simulink model "invertedPendolum"  (R2019a)
settings: Solver=VariableStepAuto  StartTime=0.0  StopTime=60  FixedStep=0.0001  RelTol=1e-4
InitFcn:
  | simulationVar
values from neighbouring files (symbols this model uses):
  tauMotMax = Ka * Id    (= 55296484.32)    [simulationVar.m]
libraries: simulink x6
settings Model: Creator=alfyhack  LastModifiedBy=alfyhack
settings SolverCC: AlgebraicLoopSolver=LineSearch
settings DebuggingCC: UnderSpecifiedDimensionMsg=warning

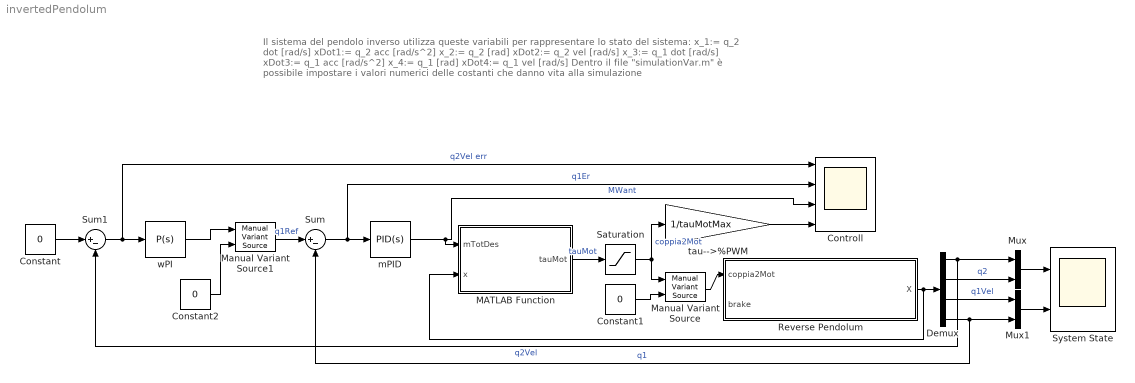
== system invertedPendolum ==
  note: Il sistema del pendolo inverso utilizza queste variabili per rappresentare lo stato del sistema:
      |
      | x_1:= q_2 dot  [rad/s]		xDot1:= q_2 acc   [rad/s^2]
      | x_2:= q_2        [rad]		xDot2:= q_2 vel    [rad/s]
      | x_3:= q_1 dot  [rad/s]		xDot3:= q_1 acc   [rad/s^2]
      | x_4:= q_1        [rad]		xDot4:= q_1 vel    [rad/s]
      |
      | Dentro il file "simulationVar.m" è possibile impostare i valori numerici delle costanti che danno vita alla simulazione
  Constant : Constant  Value=0
  Constant1 : Constant  Value=0
  Constant2 : Constant  Value=0
  Controll : Scope  NumInputPorts=4
  Demux : Demux
  MATLAB Function : MATLAB Function  TreatAsAtomicUnit=on
  Manual Variant Source : simulink/Signal Routing/Manual Variant Source  NumChoices=2  LabelModeActiveChoice=V_2
      settings: SourceProductName=Simulink
  Manual Variant Source1 : simulink/Signal Routing/Manual Variant Source  NumChoices=2  LabelModeActiveChoice=V_1
      settings: SourceProductName=Simulink
  Mux : Mux  Inputs=2
  Mux1 : Mux  Inputs=2
  Reverse Pendolum : Subsystem
  Saturation : Saturate  UpperLimit=tauMotMax  LowerLimit=-tauMotMax
  Sum : Sum  Inputs=|+-
  Sum1 : Sum  Inputs=|+-
  System State : Scope  NumInputPorts=2
  mPID : simulink/Continuous/PID Controller  Controller=PID  Form=Parallel  TimeDomain=Continuous-time  SampleTime=-1  IntegratorMethod=Forward Euler  FilterMethod=Forward Euler  ControllerParametersSource=internal  P=2418132733.30145  I=2565122053.15996  D=559751835.250899  UseFilter=on  N=123.582703784114  TunerSelectOption=Transfer Function Based (PID Tuner App)  InitialConditionSource=internal  InitialConditionForIntegrator=0  InitialConditionForFilter=0  DifferentiatorICPrevScaledInput=0  ExternalReset=none  TrackingMode=off  Kt=1  LimitOutput=off  UpperSaturationLimit=1000  LowerSaturationLimit=1000  LinearizeAsGain=off  AntiWindupMode=none  Kb=1  POutMin=[]  POutMax=[]  IOutMin=[]  IOutMax=[]  DOutMin=[]  DOutMax=[]  NOutMin=[]  NOutMax=[]  SumOutMin=[]  SumOutMax=[]  SaturationOutMin=[]  SaturationOutMax=[]  PParamMin=[]  PParamMax=[]  IParamMin=[]  IParamMax=[]  DParamMin=[]  DParamMax=[]  NParamMin=[]  NParamMax=[]  KbParamMin=[]  KbParamMax=[]  KtParamMin=[]  KtParamMax=[]  KbOutMin=[]  KbOutMax=[]  KtOutMin=[]  KtOutMax=[]  IntegratorOutMin=[]  IntegratorOutMax=[]  FilterOutMin=[]  FilterOutMax=[]  SumI1OutMin=[]  SumI1OutMax=[]  SumI2OutMin=[]  SumI2OutMax=[]  SumI3OutMin=[]  SumI3OutMax=[]  SumI4OutMin=[]  SumI4OutMax=[]  SumDOutMin=[]  SumDOutMax=[]  DifferentiatorOutMin=[]  DifferentiatorOutMax=[]  FilterDiffOutCoefMin=[]  FilterDiffOutCoefMax=[]  ReciprocalOutMin=[]  ReciprocalOutMax=[]  SumDenOutMin=[]  SumDenOutMax=[]  SumNumOutMin=[]  SumNumOutMax=[]  DivideOutMin=[]  DivideOutMax=[]  IntegratorContinuousStateAttributes=''  IntegratorStateMustResolveToSignalObject=off  IntegratorRTWStateStorageClass=Auto  FilterContinuousStateAttributes=''  FilterStateMustResolveToSignalObject=off  FilterRTWStateStorageClass=Auto  ParallelPVariant=InternalParameters  IdealPVariant=Disabled  IVariant=InternalParameters  DVariant=InternalParameters  IntegratorVariant=Continuous  SatVariant=Disabled  AWVariant=Passthrough  PCopyVariant=Disabled  TRVariant=Disabled  FdbkBlocksVariant=Forward  IdealPFdbkVariant=Disabled  SatFdbkVariant=Disabled  DerivativeFilterVariant=ContFilter  NVariant=InternalParameters  NCopyVariant=Disabled  FilterICVariant=InternalICsFilter  IntegratorICVariant=InternalICs  ExternalResetVariant=Disabled  TRSumVariant=Passthrough  SumFdbkVariant=Disabled  SumVariant=Sum_PID
  tau-->%PWM : Gain  Gain=1/tauMotMax
  wPI : simulink/Continuous/PID Controller  Controller=P  Form=Parallel  TimeDomain=Continuous-time  SampleTime=-1  IntegratorMethod=Forward Euler  FilterMethod=Forward Euler  ControllerParametersSource=internal  P=0.000223072388975436  I=0.001  D=1  UseFilter=on  N=2000  TunerSelectOption=Transfer Function Based (PID Tuner App)  InitialConditionSource=internal  InitialConditionForIntegrator=0  InitialConditionForFilter=0  DifferentiatorICPrevScaledInput=0  ExternalReset=none  TrackingMode=off  Kt=1  LimitOutput=on  UpperSaturationLimit=0.1  LowerSaturationLimit=-0.1  LinearizeAsGain=off  AntiWindupMode=none  Kb=1  POutMin=[]  POutMax=[]  IOutMin=[]  IOutMax=[]  DOutMin=[]  DOutMax=[]  NOutMin=[]  NOutMax=[]  SumOutMin=[]  SumOutMax=[]  SaturationOutMin=[]  SaturationOutMax=[]  PParamMin=[]  PParamMax=[]  IParamMin=[]  IParamMax=[]  DParamMin=[]  DParamMax=[]  NParamMin=[]  NParamMax=[]  KbParamMin=[]  KbParamMax=[]  KtParamMin=[]  KtParamMax=[]  KbOutMin=[]  KbOutMax=[]  KtOutMin=[]  KtOutMax=[]  IntegratorOutMin=[]  IntegratorOutMax=[]  FilterOutMin=[]  FilterOutMax=[]  SumI1OutMin=[]  SumI1OutMax=[]  SumI2OutMin=[]  SumI2OutMax=[]  SumI3OutMin=[]  SumI3OutMax=[]  SumI4OutMin=[]  SumI4OutMax=[]  SumDOutMin=[]  SumDOutMax=[]  DifferentiatorOutMin=[]  DifferentiatorOutMax=[]  FilterDiffOutCoefMin=[]  FilterDiffOutCoefMax=[]  ReciprocalOutMin=[]  ReciprocalOutMax=[]  SumDenOutMin=[]  SumDenOutMax=[]  SumNumOutMin=[]  SumNumOutMax=[]  DivideOutMin=[]  DivideOutMax=[]  IntegratorContinuousStateAttributes=''  IntegratorStateMustResolveToSignalObject=off  IntegratorRTWStateStorageClass=Auto  FilterContinuousStateAttributes=''  FilterStateMustResolveToSignalObject=off  FilterRTWStateStorageClass=Auto  ParallelPVariant=InternalParameters  IdealPVariant=Disabled  IVariant=Disabled  DVariant=Disabled  IntegratorVariant=Disabled  SatVariant=Enabled  AWVariant=Disabled  PCopyVariant=Disabled  TRVariant=Disabled  FdbkBlocksVariant=Forward  IdealPFdbkVariant=Disabled  SatFdbkVariant=Disabled  DerivativeFilterVariant=Disabled  NVariant=Disabled  NCopyVariant=Disabled_SignalSpec  FilterICVariant=Disabled  IntegratorICVariant=Disabled  ExternalResetVariant=Disabled  TRSumVariant=Passthrough  SumFdbkVariant=Disabled  SumVariant=Passthrough_P
  wires:
  Demux/4 -> Mux1/2, Sum/2  "q1"
  Demux/1 -> Mux/1, Sum1/2  "q2Vel"
  MATLAB Function/1(tauMot) -> Saturation/1  "tauMot"
  mPID/1 -> Controll/3, MATLAB Function/1(mTotDes)  "MWant"
  Sum/1 -> Controll/2, mPID/1  "q1Er"
  wPI/1 -> Manual Variant Source1/1
  Constant/1 -> Sum1/1
  Sum1/1 -> Controll/1, wPI/1  "q2Vel err"
  Saturation/1 -> tau-->%PWM/1, Manual Variant Source/1  "coppia2Mot"
  Reverse Pendolum/1(X) -> Demux/1, MATLAB Function/2(x)
  Demux/3 -> Mux1/1  "q1Vel"
  Demux/2 -> Mux/2  "q2"
  Mux1/1 -> System State/2
  Mux/1 -> System State/1
  tau-->%PWM/1 -> Controll/4
  Manual Variant Source/1 -> Reverse Pendolum/1(coppia2Mot)
  Constant1/1 -> Manual Variant Source/2
  Manual Variant Source1/1 -> Sum/1  "q1Ref"
  Constant2/1 -> Manual Variant Source1/2

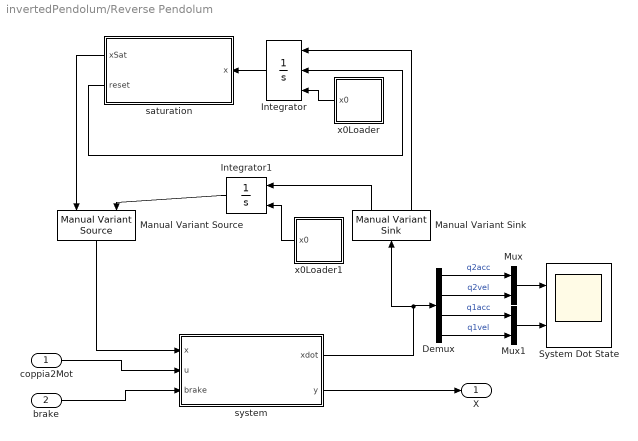
== system invertedPendolum/Reverse Pendolum ==
  coppia2Mot : Inport
  brake : Inport  Port=2
  Demux : Demux
  Integrator : Integrator  ExternalReset=rising  InitialConditionSource=external  InitialCondition=[0,0.1,0]
  Integrator1 : Integrator  InitialConditionSource=external
  Manual Variant Sink : simulink/Signal Routing/Manual Variant Sink  NumChoices=2  LabelModeActiveChoice=V_2
      settings: SourceProductName=Simulink
  Manual Variant Source : simulink/Signal Routing/Manual Variant Source  NumChoices=2  LabelModeActiveChoice=V_1
      settings: SourceProductName=Simulink
  Mux : Mux  Inputs=2
  Mux1 : Mux  Inputs=2
  System Dot State : Scope  NumInputPorts=2
  saturation : MATLAB Function  TreatAsAtomicUnit=on
  system : MATLAB Function  TreatAsAtomicUnit=on
  x0Loader : MATLAB Function  TreatAsAtomicUnit=on
  x0Loader1 : MATLAB Function  TreatAsAtomicUnit=on
  X : Outport
  wires:
  x0Loader/1(x0) -> Integrator/3
  Integrator/1 -> saturation/1(x)
  saturation/2(reset) -> Integrator/2
  coppia2Mot/1 -> system/2(u)
  system/2(y) -> X/1
  Mux/1 -> System Dot State/1
  Demux/3 -> Mux1/1  "q1acc"
  Demux/1 -> Mux/1  "q2acc"
  system/1(xdot) -> Manual Variant Sink/1, Demux/1
  Demux/2 -> Mux/2  "q2vel"
  Demux/4 -> Mux1/2  "q1vel"
  Mux1/1 -> System Dot State/2
  Manual Variant Sink/2 -> Integrator/1
  saturation/1(xSat) -> Manual Variant Source/1
  Integrator1/1 -> Manual Variant Source/2
  Manual Variant Sink/1 -> Integrator1/1
  Manual Variant Source/1 -> system/1(x)
  x0Loader1/1(x0) -> Integrator1/2
  brake/1 -> system/3(brake)

== matlab function invertedPendolum/Reverse Pendolum/system ==
  data: x input; xdot output size=4; u input; y output; brake input
function [xdot,y] = pendoloNotLinSys(x,u,brake)
%PENDOLONOTLINSYS Summary of this function goes here
% xDot1:= q2 acc    [rad/s^2]
% xDot2:= q2 vel    [rad/s]
% xDot3:= q1 acc    [rad/s^2]
% xDot4:= q1 vel    [rad/s]

% x1:= q2 dot    [rad/s]
% x2:= q2        [rad]
% x3:= q1 dot    [rad/s]
% x4:= q1        [rad]

% u:= Coppia motore [g/s^2 * mm]
% brake:= true change D2 and shutdown u

coder.extrinsic('evalin', 'assignin')

D1 = 0;                  % Needed in order to set variable class correctly
D1 = evalin('base','D1'); % Read value from workspace

Id = 0;                  % Needed in order to set variable class correctly
Id = evalin('base','Id'); % Read value from workspace

Ibtot = 0;                  % Needed in order to set variable class correctly
Ibtot = evalin('base','Ibtot'); % Read value from workspace

Kmgl = 0;                  % Needed in order to set variable class correctly
Kmgl = evalin('base','Kmgl'); % Read value from workspace

tauMotMax = 0;
tauMotMax = evalin('base','tauMotMax'); % Read value from workspace

rhoInd = 0;                  % Needed in order to set variable class correctly
rhoInd = evalin('base','rhoInd'); % Read value from workspace

rhoMec = 0;                  % Needed in order to set variable class correctly
rhoMec = evalin('base','rhoMec'); % Read value from workspace

D2 = 0;                  % Needed in order to set variable class correctly
D2 = evalin('base','D2'); % Read value from workspace

attDyn = 0;                  % Needed in order to set variable class correctly
attDyn = evalin('base','attDyn'); % Read value from workspace


% Calcoli notevoli:
% fprintf('Kmgl= %f, Ibtot=%f\t', Kmgl, Ibtot); 
skmgl = (Kmgl/Ibtot)*sin(x(4));
% fprintf('skmgl= %f\t', skmgl); 
d1friz = (D1*x(3))/Ibtot;
% fprintf('d1friz= %f\t', d1friz); 
% d2x1 = D2*x(1);
% D2 è in funzione di u, v e si ottiene moltiplicando per l'inerzia i dati
% sperimentali
% duty=abs(u/tauMotMax);
if(abs(x(1))>0.001)
%     d2x1 = (((rhoInd)*abs(u/tauMotMax)+ rhoMec)*x(1) + sign(x(1))*attDyn)*Id;
    d2x1 = ((rhoInd+rhoMec))*Id*x(1);% + sign(x(1))*attDyn;
%     d2x1 = ((rhoInd*duty+rhoMec)*x(1))*Id + sign(x(1))*attDyn;

else
    d2x1 = 0;

end
% fprintf('d2x1= %f\tduty=%f\n', d2x1,duty); 

xdot=zeros(4,1);
xdot(1) = -(1/Ibtot+1/Id)*d2x1 - skmgl + d1friz + (1/Ibtot+1/Id)*u;
xdot(2) = x(1);
xdot(3) = d2x1/Ibtot + skmgl - d1friz - u/Ibtot;
% fprintf('xdot(3)= %f\n', xdot(3));  
xdot(4) = x(3);


%per ora supponiamo di poter osservare tutto il sistema
y=x;

end

== matlab function invertedPendolum/Reverse Pendolum/saturation ==
  data: x input; xSat output; reset output
function [xSat,reset]  = phisicReaction(x)
%PHISICREACTION Summary of this function goes here
% Funzione che letto lo stato, in caso di urto con la base cambia
% in maniera realistica lo stato introducendo una saturazione.

% xDot1:= q2 acc    [rad/s^2]
% xDot2:= q2 vel    [rad/s]
% xDot3:= q1 acc    [rad/s^2]
% xDot4:= q1 vel    [rad/s]

% x1:= q2 dot    [rad/s]
% x2:= q2        [rad]
% x3:= q1 dot    [rad/s]
% x4:= q1        [rad]

coder.extrinsic('evalin', 'assignin')
q1Max = 0;                  % Needed in order to set variable class correctly
q1Max = evalin('base','q1Max'); % Read value from workspace

xSat=x;
if((abs(x(4))>q1Max)&&(sign(x(3))==sign(x(4))))
    xSat(3)=-x(3)*0.1;          % dissipazione di energia
    xSat(4)=sign(x(4))*(q1Max*0.99999);   % riposizionamento
    
    %to reset integrator state
    assignin('base','x0',xSat); % Assign value back to workspace
    reset=1;
else
    reset=0;
end

end

== matlab function invertedPendolum/Reverse Pendolum/x0Loader ==
  data: x0 output
function x0 = loadX0()
% xDot1:= q2 acc    [rad/s^2]
% xDot2:= q2 vel    [rad/s]
% xDot3:= q1 acc    [rad/s^2]
% xDot4:= q1 vel    [rad/s]

% x1:= q2 dot    [rad/s]
% x2:= q2        [rad]
% x3:= q1 dot    [rad/s]
% x4:= q1        [rad]
coder.extrinsic('evalin', 'assignin')
x0 = zeros(4,1);          % Needed in order to set variable class correctly
x0 = evalin('base','x0'); % Read value from workspace

== matlab function invertedPendolum/Reverse Pendolum/x0Loader1 ==
  data: x0 output
function x0 = loadX0()
% xDot1:= q2 acc    [rad/s^2]
% xDot2:= q2 vel    [rad/s]
% xDot3:= q1 acc    [rad/s^2]
% xDot4:= q1 vel    [rad/s]

% x1:= q2 dot    [rad/s]
% x2:= q2        [rad]
% x3:= q1 dot    [rad/s]
% x4:= q1        [rad]
coder.extrinsic('evalin', 'assignin')
x0 = zeros(4,1);          % Needed in order to set variable class correctly
x0 = evalin('base','x0'); % Read value from workspace

== matlab function invertedPendolum/MATLAB Function ==
  data: mTotDes input; x input; tauMot output size=1
function tauMot = Mwant(mTotDes, x)
% x1:= q2 dot    [rad/s]
% x2:= q2        [rad]
% x3:= q1 dot    [rad/s]
% x4:= q1        [rad]
% tauMot:= Coppia motore [g/s^2 * mm]

coder.extrinsic('evalin', 'assignin')
Kmgl = 0;                  % Needed in order to set variable class correctly
Kmgl = evalin('base','Kmgl'); % Read value from workspace

D1 = 0;                  % Needed in order to set variable class correctly
D1 = evalin('base','D1'); % Read value from workspace

% D2 = 0;                  % Needed in order to set variable class correctly
% D2 = evalin('base','D2'); % Read value from workspace

tauMotMax = 0;           % Needed in order to set variable class correctly
tauMotMax = evalin('base','tauMotMax'); % Read value from workspace

Id = 0;                  % Needed in order to set variable class correctly
Id = evalin('base','Id'); % Read value from workspace


rhoInd = 0;                  % Needed in order to set variable class correctly
rhoInd = evalin('base','rhoInd'); % Read value from workspace

rhoMec = 0;                  % Needed in order to set variable class correctly
rhoMec = evalin('base','rhoMec'); % Read value from workspace

attDyn = 0;                  % Needed in order to set variable class correctly
attDyn = evalin('base','attDyn'); % Read value from workspace

% Frenata del motore in funzione della velocità
% d2x1 = (((rhoInd) *abs(u/tauMotMax) + rhoMec)*x(1) + sign(x(1))*uDym)*Id;

% d2x1 = (((rhoInd) + rhoMec)*x(1) + sign(x(1))*uDym)*Id;
% duty=abs(u/tauMotMax);
if(abs(x(1))>0.001)
%     d2x1 = (((rhoInd)*abs(u/tauMotMax)+ rhoMec)*x(1) + sign(x(1))*attDyn)*Id;
    d2x1 = ((rhoInd+rhoMec))*Id*x(1);% + sign(x(1))*attDyn;
%     d2x1 = ((rhoInd*duty+rhoMec)*x(1))*Id + sign(x(1))*attDyn;

else
    d2x1 = 0;

end

% fprintf("d2x1=%f\n",d2x1);

tauMot = -mTotDes + d2x1 + Kmgl*sin(x(4)) - D1*x(3);
% fprintf("tauMot=%f\n",tauMot);
end
